simulink model "CDMA1_sim_TxRx_2020"  (R2016a)
settings: Solver=ode45  StartTime=0.0  StopTime=20  MaxStep=.01  MinStep=.001  RelTol=1e-3
libraries: commseqgen2 x4, dsparch4 x2
settings Model: Creator=user  LastModifiedBy=Simona
settings DataIOCC: LimitDataPoints=on  SaveFormat=Array  SignalLoggingSaveFormat=ModelDataLogs
settings OptimizationCC: ExpressionDepthLimit=2147483647  InitFltsAndDblsToZero=on
settings DebuggingCC: SaveWithParameterizedLinksMsg=none  UnderspecifiedInitializationDetection=Classic  MergeDetectMultiDrivingBlocksExec=none  SolverPrmCheckMsg=warning  MultiTaskCondExecSysMsg=none  FcnCallInpInsideContextMsg=UseLocalSettings  StateNameClashWarn=warning
settings HardwareCC: ProdBitPerPointer=32  ProdLargestAtomicFloat=None  ProdIntDivRoundTo=Undefined  ProdEndianess=Unspecified  ProdWordSize=32  ProdHWDeviceType=32-bit Generic
settings ModelReferenceCC: PropagateSignalLabelsOutOfModel=off
settings GRTTargetCC: CombineOutputUpdateFcns=off  GRTInterface=on
settings ConfigComp: CovModelRefEnable=Off

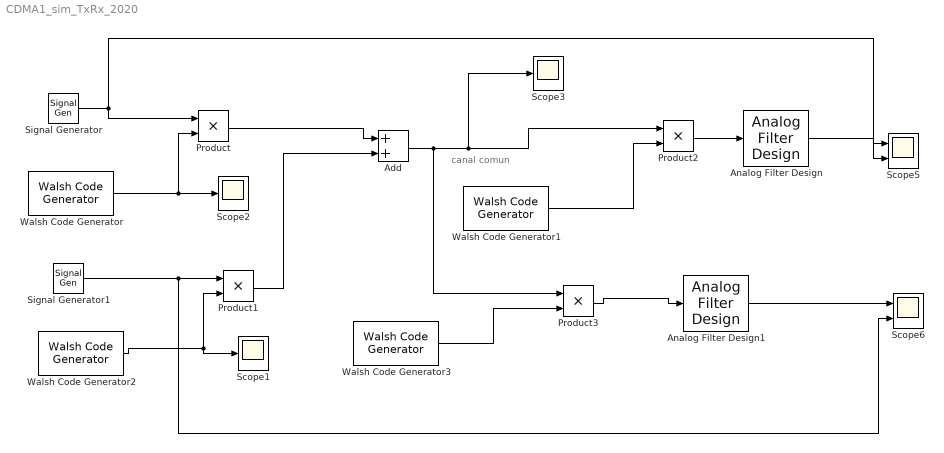
== system CDMA1_sim_TxRx_2020 ==
  note: canal comun
  Add : Sum
  Analog Filter Design : dsparch4/Analog Filter Design  method=Butterworth  filttype=Lowpass  N=10  Wlo=2*2*pi  Whi=80  Rp=2  Rs=40
  Analog Filter Design1 : dsparch4/Analog Filter Design  method=Butterworth  filttype=Lowpass  N=10  Wlo=5*2*pi  Whi=80  Rp=2  Rs=40
  Product{,1..3} (4 alike) : Product  RndMeth=Zero
  Scope1 : Scope
  Scope2 : Scope
  Scope3 : Scope
  Scope5 : Scope  NumInputPorts=2
  Scope6 : Scope  NumInputPorts=2
  Signal Generator : SignalGenerator
  Signal Generator1 : SignalGenerator  WaveForm=sawtooth  Frequency=2
  Walsh Code Generator : commseqgen2/Walsh Code Generator  length=64  index=2  ts=1/64  frameBased=off  sampPerFrame=1  outDataType=double
  Walsh Code Generator1 : commseqgen2/Walsh Code Generator  length=64  index=2  ts=1/64  frameBased=off  sampPerFrame=1  outDataType=double
  Walsh Code Generator2 : commseqgen2/Walsh Code Generator  length=64  index=32  ts=1/64  frameBased=off  sampPerFrame=1  outDataType=double
  Walsh Code Generator3 : commseqgen2/Walsh Code Generator  length=64  index=32  ts=1/64  frameBased=off  sampPerFrame=1  outDataType=double
  wires:
  Signal Generator/1 -> Scope5/2, Product/1
  Walsh Code Generator/1 -> Product/2, Scope2/1
  Product/1 -> Add/1
  Signal Generator1/1 -> Product1/1, Scope6/2
  Walsh Code Generator2/1 -> Product1/2, Scope1/1
  Walsh Code Generator1/1 -> Product2/2
  Add/1 -> Product2/1, Scope3/1, Product3/1
  Walsh Code Generator3/1 -> Product3/2
  Product2/1 -> Analog Filter Design/1
  Product3/1 -> Analog Filter Design1/1
  Analog Filter Design/1 -> Scope5/1
  Product1/1 -> Add/2
  Analog Filter Design1/1 -> Scope6/1
